simulink model "PSAS_Rocket_sim"  (R2013a)
settings: Solver=ode45  StartTime=0.0  StopTime=10.0  RelTol=1e-3
values from neighbouring files (symbols this model uses):
  burn = 0.25    [PSAS_Rocket_sys.m]    (also in stevens_state_space_for_rocket.m)
  burntime = m_fuel/burn    (= 40)    [PSAS_Rocket_sys.m]    (also in stevens_state_space_for_rocket.m = 76)
  F_pitch = 5.5    [PSAS_Rocket_sys.m]
  F_roll = 7    [PSAS_Rocket_sys.m]
  F_yaw = 5.5    [PSAS_Rocket_sys.m]
  g = 9.81    [PSAS_Rocket_sys.m]    (also in stevens_state_space_for_rocket.m)
  hz = 5    [PSAS_Rocket_sys.m]    (also in roll_sys.m; rotational_system.m = 10)
  Inertia = [Ixx -Ixy -Ixz; -Ixy Iyy -Iyz; -Ixz -Iyz Izz]    [PSAS_Rocket_sys.m]
  Ixx = .05    (= 0.05)    [PSAS_Rocket_sys.m]
  Ixy = 0.02    [PSAS_Rocket_sys.m]
  Ixz = 0.05    [PSAS_Rocket_sys.m]
  Iyy = .05    (= 0.05)    [PSAS_Rocket_sys.m]
  Iyz = 0.02    [PSAS_Rocket_sys.m]
  Izz = 0.0169    [PSAS_Rocket_sys.m]
  kp_phi = .001    (= 0.001)    [PSAS_Rocket_sys.m]
  kp_psi = .2    (= 0.2)    [PSAS_Rocket_sys.m]
  kp_theta = .001    (= 0.001)    [PSAS_Rocket_sys.m]
  m_fuel = 10    [PSAS_Rocket_sys.m]    (also in stevens_state_space_for_rocket.m = 19)
  m_inst = 3    [PSAS_Rocket_sys.m]    (also in stevens_state_space_for_rocket.m = 3.8)
  q1 = cos(psi/2)*cos(theta/2)*cos(phi/2)     + sin(psi/2)*sin(theta/2)*sin(phi/2)    [PSAS_Rocket_sys.m]    (also in stevens_state_space_for_rocket.m = sin(phi/2)*cos(theta/2)*cos(psi/2)-cos(phi/2)*     sin(theta)
  q2 = cos(psi/2)*cos(theta/2)*sin(phi/2)     - sin(psi/2)*sin(theta/2)*cos(phi/2)    [PSAS_Rocket_sys.m]    (also in stevens_state_space_for_rocket.m = cos(phi/2)*sin(theta/2)*cos(psi/2)+sin(phi/2)*     cos(theta)
  q3 = cos(psi/2)*sin(theta/2)*cos(phi/2)     + sin(psi/2)*cos(theta/2)*sin(phi/2)    [PSAS_Rocket_sys.m]    (also in stevens_state_space_for_rocket.m = cos(phi/2)*cos(theta/2)*sin(psi/2)-sin(phi/2)*     sin(theta)
  q4 = sin(psi/2)*cos(theta/2)*cos(phi/2)     - cos(psi/2)*sin(theta/2)*sin(phi/2)    [PSAS_Rocket_sys.m]
  roll_disturbance = 1*pi/180    (= 0.0174532925199)    [PSAS_Rocket_sys.m]
  tau = 0.02    [PSAS_Rocket_sys.m]    (also in lqrQfinder.m = 0.009; stevens_state_space_for_rocket.m = 0.05)
  theta_in = 90*pi/180    (= 1.57079632679)    [PSAS_Rocket_sys.m]
  theta_in_ramp = 2    [PSAS_Rocket_sys.m]
  thrust = 4440.8    [PSAS_Rocket_sys.m]    (also in stevens_state_space_for_rocket.m = 444.8)
  thrust_lag = 1.5    [PSAS_Rocket_sys.m]
  ts = .003    (= 0.003)    [PSAS_Rocket_sys.m]    (also in stevens_state_space_for_rocket.m = 0.01)
libraries: simulink x8
settings Model: Creator=kenny  LastModifiedBy=kenny

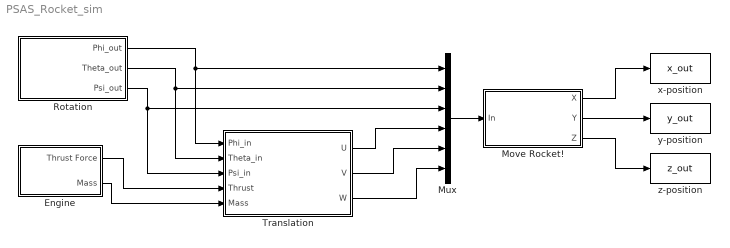
== system PSAS_Rocket_sim ==
  Engine : Subsystem
  Move Rocket! : Subsystem
  Mux : Mux  Inputs=6
  Rotation : Subsystem
  Translation : Subsystem
  x-position : ToWorkspace  VariableName=x_out  SampleTime=-1  SaveFormat=Structure With Time
  y-position : ToWorkspace  VariableName=y_out  SampleTime=-1  SaveFormat=Structure With Time
  z-position : ToWorkspace  VariableName=z_out  SampleTime=-1  SaveFormat=Structure With Time
  wires:
  Rotation/1(Phi_out) -> Translation/1(Phi_in), Mux/1
  Rotation/2(Theta_out) -> Translation/2(Theta_in), Mux/2
  Rotation/3(Psi_out) -> Translation/3(Psi_in), Mux/3
  Translation/2(V) -> Mux/5
  Translation/3(W) -> Mux/6
  Translation/1(U) -> Mux/4
  Engine/1(Thrust Force) -> Translation/4(Thrust)
  Engine/2(Mass) -> Translation/5(Mass)
  Mux/1 -> Move Rocket!/1(In)
  Move Rocket!/2(Y) -> y-position/1
  Move Rocket!/1(X) -> x-position/1
  Move Rocket!/3(Z) -> z-position/1

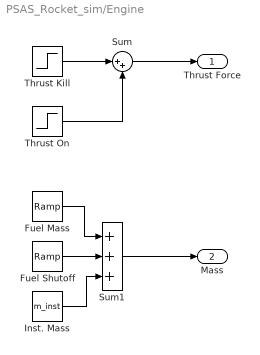
== system PSAS_Rocket_sim/Engine ==
  Fuel Mass : simulink/Sources/Ramp  slope=-burn  start=0  X0=m_fuel
  Fuel Shutoff : simulink/Sources/Ramp  slope=burn  start=burntime  X0=0
  Inst. Mass : Constant  Value=m_inst
  Sum : Sum  Inputs=|++
  Sum1 : Sum  Inputs=+++
  Thrust Kill : Step  Time=burntime+thrust_lag  After=-thrust  SampleTime=0
  Thrust On : Step  Time=thrust_lag  After=thrust  SampleTime=0
  Thrust Force : Outport
  Mass : Outport  Port=2
  wires:
  Thrust Kill/1 -> Sum/1
  Thrust On/1 -> Sum/2
  Sum/1 -> Thrust Force/1
  Sum1/1 -> Mass/1
  Fuel Mass/1 -> Sum1/1
  Fuel Shutoff/1 -> Sum1/2
  Inst. Mass/1 -> Sum1/3

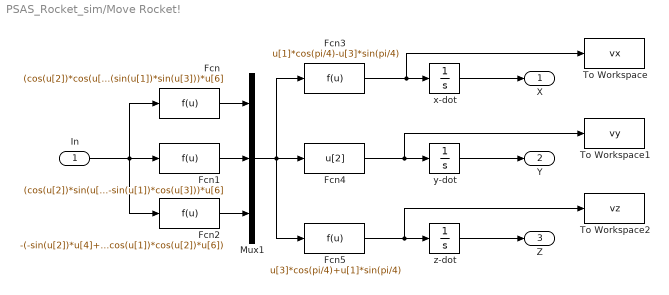
== system PSAS_Rocket_sim/Move Rocket! ==
  In : Inport
  Fcn : Fcn  Expr=(cos(u[2])*cos(u[3]))*u[4]+(sin(u[1])*sin(u[2])*cos(u[3])-cos(u[1])*sin(u[3]))*u[5]+(sin(u[1])*sin(u[3]))*u[6]
  Fcn1 : Fcn  Expr=(cos(u[2])*sin(u[3]))*u[4]+(sin(u[1])*sin(u[2])*sin(u[3])+cos(u[1])*cos(u[3]))*u[5]+(cos(u[1])*sin(u[2])*sin(u[3])-sin(u[1])*cos(u[3]))*u[6]
  Fcn2 : Fcn  Expr=-(-sin(u[2])*u[4]+sin(u[1])*cos(u[2])*u[5]+cos(u[1])*cos(u[2])*u[6])
  Fcn3 : Fcn  Expr=u[1]*cos(pi/4)-u[3]*sin(pi/4)
  Fcn4 : Fcn  Expr=u[2]
  Fcn5 : Fcn  Expr=u[3]*cos(pi/4)+u[1]*sin(pi/4)
  Mux1 : Mux  Inputs=3
  To Workspace : ToWorkspace  VariableName=vx  SampleTime=-1
  To Workspace1 : ToWorkspace  VariableName=vy  SampleTime=-1
  To Workspace2 : ToWorkspace  VariableName=vz  SampleTime=-1
  x-dot : Integrator
  y-dot : Integrator
  z-dot : Integrator
  X : Outport
  Y : Outport  Port=2
  Z : Outport  Port=3
  wires:
  In/1 -> Fcn/1, Fcn2/1, Fcn1/1
  z-dot/1 -> Z/1
  y-dot/1 -> Y/1
  x-dot/1 -> X/1
  Fcn/1 -> Mux1/1
  Fcn1/1 -> Mux1/2
  Fcn2/1 -> Mux1/3
  Mux1/1 -> Fcn4/1, Fcn3/1, Fcn5/1
  Fcn3/1 -> To Workspace/1, x-dot/1
  Fcn4/1 -> y-dot/1, To Workspace1/1
  Fcn5/1 -> z-dot/1, To Workspace2/1

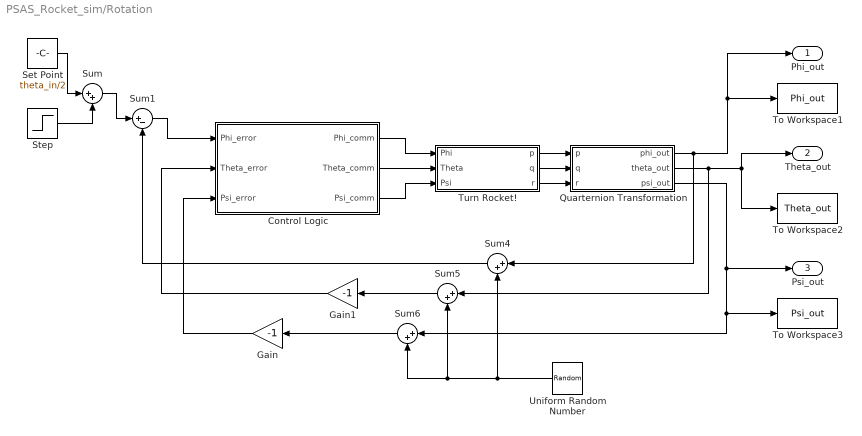
== system PSAS_Rocket_sim/Rotation ==
  Control Logic : Subsystem
  Gain : Gain  Gain=-1
  Gain1 : Gain  Gain=-1
  Quarternion Transformation : Subsystem
  Set Point : Constant  Value=theta_in/2
  Step : Step  Time=theta_in_ramp  After=theta_in/2  SampleTime=0
  Sum{,4..6} (4 alike) : Sum  Inputs=|++
  Sum1 : Sum  Inputs=|+-
  To Workspace1 : ToWorkspace  VariableName=Phi_out  SampleTime=-1  SaveFormat=Structure With Time
  To Workspace2 : ToWorkspace  VariableName=Theta_out  SampleTime=-1  SaveFormat=Structure With Time
  To Workspace3 : ToWorkspace  VariableName=Psi_out  SampleTime=-1  SaveFormat=Structure With Time
  Turn Rocket! : Subsystem
  Uniform Random Number : UniformRandomNumber  Minimum=-roll_disturbance  Maximum=roll_disturbance  SampleTime=ts
  Phi_out : Outport
  Theta_out : Outport  Port=2
  Psi_out : Outport  Port=3
  wires:
  Step/1 -> Sum/2
  Set Point/1 -> Sum/1
  Sum/1 -> Sum1/1
  Control Logic/1(Phi_comm) -> Turn Rocket!/1(Phi)
  Control Logic/2(Theta_comm) -> Turn Rocket!/2(Theta)
  Control Logic/3(Psi_comm) -> Turn Rocket!/3(Psi)
  Turn Rocket!/1(p) -> Quarternion Transformation/1(p)
  Turn Rocket!/2(q) -> Quarternion Transformation/2(q)
  Turn Rocket!/3(r) -> Quarternion Transformation/3(r)
  Quarternion Transformation/2(theta_out) -> Sum5/1, To Workspace2/1, Theta_out/1
  Quarternion Transformation/1(phi_out) -> Sum4/1, Phi_out/1, To Workspace1/1
  Quarternion Transformation/3(psi_out) -> Sum6/1, To Workspace3/1, Psi_out/1
  Uniform Random Number/1 -> Sum6/2, Sum5/2, Sum4/2
  Sum6/1 -> Gain/1
  Sum5/1 -> Gain1/1
  Gain/1 -> Control Logic/3(Psi_error)
  Gain1/1 -> Control Logic/2(Theta_error)
  Sum1/1 -> Control Logic/1(Phi_error)
  Sum4/1 -> Sum1/2

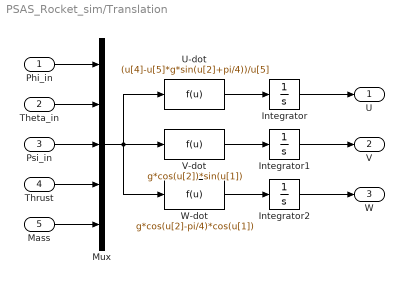
== system PSAS_Rocket_sim/Translation ==
  Phi_in : Inport
  Theta_in : Inport  Port=2
  Psi_in : Inport  Port=3
  Thrust : Inport  Port=4
  Mass : Inport  Port=5
  Integrator : Integrator
  Integrator1 : Integrator
  Integrator2 : Integrator
  Mux : Mux  Inputs=5
  U-dot : Fcn  Expr=(u[4]-u[5]*g*sin(u[2]+pi/4))/u[5]
  V-dot : Fcn  Expr=g*cos(u[2])*sin(u[1])
  W-dot : Fcn  Expr=g*cos(u[2]-pi/4)*cos(u[1])
  U : Outport
  V : Outport  Port=2
  W : Outport  Port=3
  wires:
  Phi_in/1 -> Mux/1
  Theta_in/1 -> Mux/2
  Psi_in/1 -> Mux/3
  U-dot/1 -> Integrator/1
  Mux/1 -> U-dot/1, V-dot/1, W-dot/1
  V-dot/1 -> Integrator1/1
  W-dot/1 -> Integrator2/1
  Thrust/1 -> Mux/4
  Mass/1 -> Mux/5
  Integrator/1 -> U/1
  Integrator1/1 -> V/1
  Integrator2/1 -> W/1

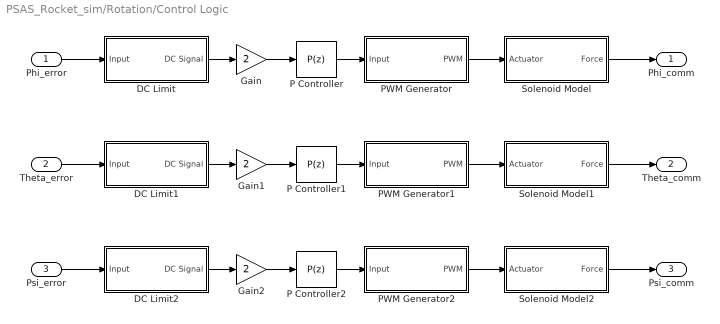
== system PSAS_Rocket_sim/Rotation/Control Logic ==
  Phi_error : Inport
  Theta_error : Inport  Port=2
  Psi_error : Inport  Port=3
  DC Limit : Subsystem
  DC Limit1 : Subsystem
  DC Limit2 : Subsystem
  Gain : Gain  Gain=2
  Gain1 : Gain  Gain=2
  Gain2 : Gain  Gain=2
  P Controller : simulink/Continuous/PID Controller  Controller=P  TimeDomain=Discrete-time  SampleTime=ts  IntegratorMethod=Forward Euler  FilterMethod=Forward Euler  Form=Parallel  P=kp_phi  I=0  D=0  N=100  InitialConditionSource=internal  InitialConditionForIntegrator=0  InitialConditionForFilter=0  ExternalReset=none  LimitOutput=off  UpperSaturationLimit=inf  LowerSaturationLimit=-inf  LinearizeAsGain=on  AntiWindupMode=none  Kb=1  TrackingMode=off  Kt=1  PParamMin=[]  PParamMax=[]  IParamMin=[]  IParamMax=[]  DParamMin=[]  DParamMax=[]  NParamMin=[]  NParamMax=[]  KbParamMin=[]  KbParamMax=[]  KtParamMin=[]  KtParamMax=[]  POutMin=[]  POutMax=[]  IOutMin=[]  IOutMax=[]  DOutMin=[]  DOutMax=[]  NOutMin=[]  NOutMax=[]  KbOutMin=[]  KbOutMax=[]  KtOutMin=[]  KtOutMax=[]  IntegratorOutMin=[]  IntegratorOutMax=[]  FilterOutMin=[]  FilterOutMax=[]  SumOutMin=[]  SumOutMax=[]  SumI1OutMin=[]  SumI1OutMax=[]  SumI2OutMin=[]  SumI2OutMax=[]  SumI3OutMin=[]  SumI3OutMax=[]  SumDOutMin=[]  SumDOutMax=[]  SaturationOutMin=[]  SaturationOutMax=[]  IntegratorContinuousStateAttributes=''  IntegratorStateMustResolveToSignalObject=off  IntegratorRTWStateStorageClass=Auto  FilterContinuousStateAttributes=''  FilterStateMustResolveToSignalObject=off  FilterRTWStateStorageClass=Auto
  P Controller1 : simulink/Continuous/PID Controller  Controller=P  TimeDomain=Discrete-time  SampleTime=ts  IntegratorMethod=Forward Euler  FilterMethod=Forward Euler  Form=Parallel  P=kp_theta  I=0  D=0  N=100  InitialConditionSource=internal  InitialConditionForIntegrator=0  InitialConditionForFilter=0  ExternalReset=none  LimitOutput=off  UpperSaturationLimit=inf  LowerSaturationLimit=-inf  LinearizeAsGain=on  AntiWindupMode=none  Kb=1  TrackingMode=off  Kt=1  PParamMin=[]  PParamMax=[]  IParamMin=[]  IParamMax=[]  DParamMin=[]  DParamMax=[]  NParamMin=[]  NParamMax=[]  KbParamMin=[]  KbParamMax=[]  KtParamMin=[]  KtParamMax=[]  POutMin=[]  POutMax=[]  IOutMin=[]  IOutMax=[]  DOutMin=[]  DOutMax=[]  NOutMin=[]  NOutMax=[]  KbOutMin=[]  KbOutMax=[]  KtOutMin=[]  KtOutMax=[]  IntegratorOutMin=[]  IntegratorOutMax=[]  FilterOutMin=[]  FilterOutMax=[]  SumOutMin=[]  SumOutMax=[]  SumI1OutMin=[]  SumI1OutMax=[]  SumI2OutMin=[]  SumI2OutMax=[]  SumI3OutMin=[]  SumI3OutMax=[]  SumDOutMin=[]  SumDOutMax=[]  SaturationOutMin=[]  SaturationOutMax=[]  IntegratorContinuousStateAttributes=''  IntegratorStateMustResolveToSignalObject=off  IntegratorRTWStateStorageClass=Auto  FilterContinuousStateAttributes=''  FilterStateMustResolveToSignalObject=off  FilterRTWStateStorageClass=Auto
  P Controller2 : simulink/Continuous/PID Controller  Controller=P  TimeDomain=Discrete-time  SampleTime=ts  IntegratorMethod=Forward Euler  FilterMethod=Forward Euler  Form=Parallel  P=kp_psi  I=0  D=0  N=100  InitialConditionSource=internal  InitialConditionForIntegrator=0  InitialConditionForFilter=0  ExternalReset=none  LimitOutput=off  UpperSaturationLimit=inf  LowerSaturationLimit=-inf  LinearizeAsGain=on  AntiWindupMode=none  Kb=1  TrackingMode=off  Kt=1  PParamMin=[]  PParamMax=[]  IParamMin=[]  IParamMax=[]  DParamMin=[]  DParamMax=[]  NParamMin=[]  NParamMax=[]  KbParamMin=[]  KbParamMax=[]  KtParamMin=[]  KtParamMax=[]  POutMin=[]  POutMax=[]  IOutMin=[]  IOutMax=[]  DOutMin=[]  DOutMax=[]  NOutMin=[]  NOutMax=[]  KbOutMin=[]  KbOutMax=[]  KtOutMin=[]  KtOutMax=[]  IntegratorOutMin=[]  IntegratorOutMax=[]  FilterOutMin=[]  FilterOutMax=[]  SumOutMin=[]  SumOutMax=[]  SumI1OutMin=[]  SumI1OutMax=[]  SumI2OutMin=[]  SumI2OutMax=[]  SumI3OutMin=[]  SumI3OutMax=[]  SumDOutMin=[]  SumDOutMax=[]  SaturationOutMin=[]  SaturationOutMax=[]  IntegratorContinuousStateAttributes=''  IntegratorStateMustResolveToSignalObject=off  IntegratorRTWStateStorageClass=Auto  FilterContinuousStateAttributes=''  FilterStateMustResolveToSignalObject=off  FilterRTWStateStorageClass=Auto
  PWM Generator : Subsystem
  PWM Generator1 : Subsystem
  PWM Generator2 : Subsystem
  Solenoid Model : Subsystem
  Solenoid Model1 : Subsystem
  Solenoid Model2 : Subsystem
  Phi_comm : Outport
  Theta_comm : Outport  Port=2
  Psi_comm : Outport  Port=3
  wires:
  PWM Generator/1(PWM) -> Solenoid Model/1(Actuator)
  P Controller/1 -> PWM Generator/1(Input)
  Solenoid Model/1(Force) -> Phi_comm/1
  PWM Generator1/1(PWM) -> Solenoid Model1/1(Actuator)
  P Controller1/1 -> PWM Generator1/1(Input)
  Solenoid Model1/1(Force) -> Theta_comm/1
  PWM Generator2/1(PWM) -> Solenoid Model2/1(Actuator)
  P Controller2/1 -> PWM Generator2/1(Input)
  Solenoid Model2/1(Force) -> Psi_comm/1
  Phi_error/1 -> DC Limit/1(Input)
  Theta_error/1 -> DC Limit1/1(Input)
  Psi_error/1 -> DC Limit2/1(Input)
  DC Limit/1(DC Signal) -> Gain/1
  Gain/1 -> P Controller/1
  DC Limit1/1(DC Signal) -> Gain1/1
  Gain1/1 -> P Controller1/1
  DC Limit2/1(DC Signal) -> Gain2/1
  Gain2/1 -> P Controller2/1

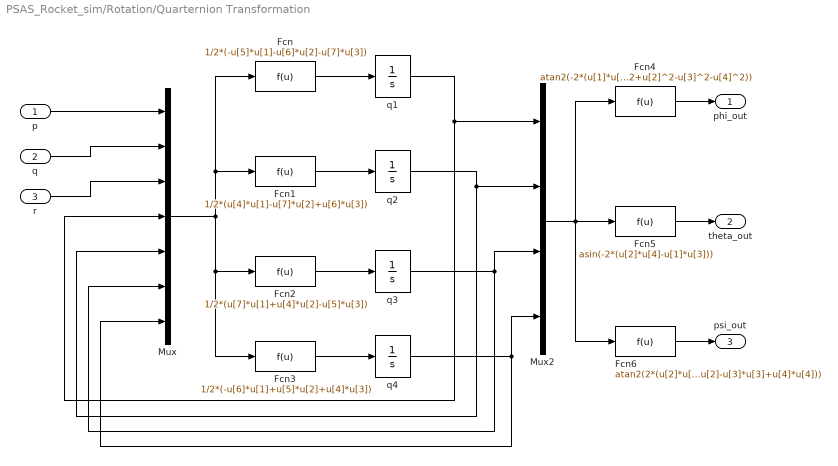
== system PSAS_Rocket_sim/Rotation/Quarternion Transformation ==
  p : Inport
  q : Inport  Port=2
  r : Inport  Port=3
  Fcn : Fcn  Expr=1/2*(-u[5]*u[1]-u[6]*u[2]-u[7]*u[3])
  Fcn1 : Fcn  Expr=1/2*(u[4]*u[1]-u[7]*u[2]+u[6]*u[3])
  Fcn2 : Fcn  Expr=1/2*(u[7]*u[1]+u[4]*u[2]-u[5]*u[3])
  Fcn3 : Fcn  Expr=1/2*(-u[6]*u[1]+u[5]*u[2]+u[4]*u[3])
  Fcn4 : Fcn  Expr=atan2(-2*(u[1]*u[2]+u[3]*u[4]),(u[1]^2+u[2]^2-u[3]^2-u[4]^2))
  Fcn5 : Fcn  Expr=asin(-2*(u[2]*u[4]-u[1]*u[3]))
  Fcn6 : Fcn  Expr=atan2(2*(u[2]*u[3]+u[1]*u[4]),(u[1]*u[1]-u[2]*u[2]-u[3]*u[3]+u[4]*u[4]))
  Mux : Mux  Inputs=7
  Mux2 : Mux
  q1 : Integrator  InitialCondition=q1
  q2 : Integrator  InitialCondition=q2
  q3 : Integrator  InitialCondition=q3
  q4 : Integrator  InitialCondition=q4
  phi_out : Outport
  theta_out : Outport  Port=2
  psi_out : Outport  Port=3
  wires:
  p/1 -> Mux/1
  q/1 -> Mux/2
  r/1 -> Mux/3
  q1/1 -> Mux/4, Mux2/1
  q2/1 -> Mux/5, Mux2/2
  q3/1 -> Mux2/3, Mux/6
  q4/1 -> Mux2/4, Mux/7
  Mux/1 -> Fcn/1, Fcn1/1, Fcn3/1, Fcn2/1
  Fcn/1 -> q1/1
  Fcn1/1 -> q2/1
  Fcn2/1 -> q3/1
  Fcn3/1 -> q4/1
  Mux2/1 -> Fcn6/1, Fcn5/1, Fcn4/1
  Fcn4/1 -> phi_out/1
  Fcn5/1 -> theta_out/1
  Fcn6/1 -> psi_out/1

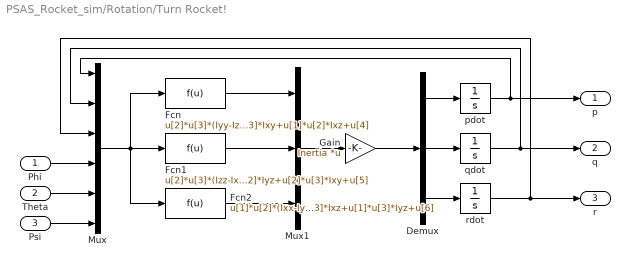
== system PSAS_Rocket_sim/Rotation/Turn Rocket! ==
  Phi : Inport
  Theta : Inport  Port=2
  Psi : Inport  Port=3
  Demux : Demux  Outputs=3
  Fcn : Fcn  Expr=u[2]*u[3]*(Iyy-Izz)+(u[2]^2-u[3]^2)*Iyz-u[1]*u[3]*Ixy+u[1]*u[2]*Ixz+u[4]
  Fcn1 : Fcn  Expr=u[2]*u[3]*(Izz-Ixx)+(u[3]^2-u[1]^2)*Ixz-u[1]*u[2]*Iyz+u[2]*u[3]*Ixy+u[5]
  Fcn2 : Fcn  Expr=u[1]*u[2]*(Ixx-Iyy)+(u[1]^2-u[2]^2)*Ixy-u[2]*u[3]*Ixz+u[1]*u[3]*Iyz+u[6]
  Gain : Gain  Gain=Inertia  Multiplication=Matrix(K*u)
  Mux : Mux  Inputs=6
  Mux1 : Mux  Inputs=3
  pdot : Integrator
  qdot : Integrator
  rdot : Integrator
  p : Outport
  q : Outport  Port=2
  r : Outport  Port=3
  wires:
  rdot/1 -> r/1, Mux/3
  qdot/1 -> q/1, Mux/2
  pdot/1 -> p/1, Mux/1
  Phi/1 -> Mux/4
  Theta/1 -> Mux/5
  Demux/1 -> pdot/1
  Demux/2 -> qdot/1
  Demux/3 -> rdot/1
  Gain/1 -> Demux/1
  Mux1/1 -> Gain/1
  Fcn/1 -> Mux1/1
  Fcn1/1 -> Mux1/2
  Fcn2/1 -> Mux1/3
  Mux/1 -> Fcn1/1, Fcn/1, Fcn2/1
  Psi/1 -> Mux/6

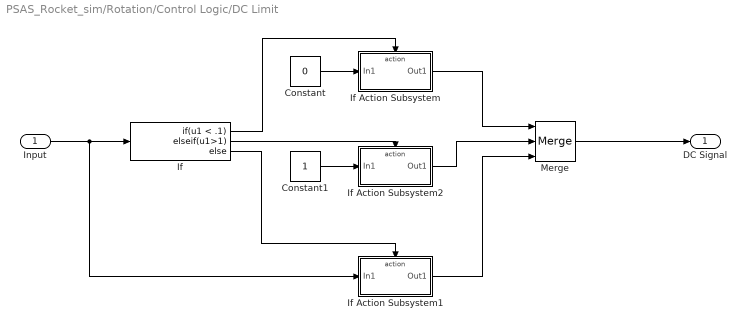
== system PSAS_Rocket_sim/Rotation/Control Logic/DC Limit ==
  Input : Inport
  Constant : Constant  Value=0
  Constant1 : Constant
  If : If  IfExpression=u1 < .1  ElseIfExpressions=u1>1
  If Action Subsystem : Subsystem  TreatAsAtomicUnit=on
  If Action Subsystem1 : Subsystem  TreatAsAtomicUnit=on
  If Action Subsystem2 : Subsystem  TreatAsAtomicUnit=on
  Merge : Merge  Inputs=3
  DC Signal : Outport
  wires:
  Input/1 -> If Action Subsystem1/1(In1), If/1
  Merge/1 -> DC Signal/1
  If Action Subsystem/1(Out1) -> Merge/1
  Constant/1 -> If Action Subsystem/1(In1)
  If/1 -> If Action Subsystem/Action
  If/3 -> If Action Subsystem1/Action
  If Action Subsystem1/1(Out1) -> Merge/3
  If/2 -> If Action Subsystem2/Action
  If Action Subsystem2/1(Out1) -> Merge/2
  Constant1/1 -> If Action Subsystem2/1(In1)

== system PSAS_Rocket_sim/Rotation/Control Logic/DC Limit1 ==
  Input : Inport
  Constant : Constant  Value=0
  Constant1 : Constant
  If : If  IfExpression=u1 < .1  ElseIfExpressions=u1>1
  If Action Subsystem : Subsystem  TreatAsAtomicUnit=on
  If Action Subsystem1 : Subsystem  TreatAsAtomicUnit=on
  If Action Subsystem2 : Subsystem  TreatAsAtomicUnit=on
  Merge : Merge  Inputs=3
  DC Signal : Outport
  wires:
  Constant1/1 -> If Action Subsystem2/1(In1)
  If Action Subsystem2/1(Out1) -> Merge/2
  If/2 -> If Action Subsystem2/Action
  If Action Subsystem1/1(Out1) -> Merge/3
  If/3 -> If Action Subsystem1/Action
  If/1 -> If Action Subsystem/Action
  Constant/1 -> If Action Subsystem/1(In1)
  If Action Subsystem/1(Out1) -> Merge/1
  Merge/1 -> DC Signal/1
  Input/1 -> If/1, If Action Subsystem1/1(In1)

== system PSAS_Rocket_sim/Rotation/Control Logic/DC Limit2 ==
  Input : Inport
  Constant : Constant  Value=0
  Constant1 : Constant
  If : If  IfExpression=u1 < .1  ElseIfExpressions=u1>1
  If Action Subsystem : Subsystem  TreatAsAtomicUnit=on
  If Action Subsystem1 : Subsystem  TreatAsAtomicUnit=on
  If Action Subsystem2 : Subsystem  TreatAsAtomicUnit=on
  Merge : Merge  Inputs=3
  DC Signal : Outport
  wires:
  Input/1 -> If Action Subsystem1/1(In1), If/1
  Merge/1 -> DC Signal/1
  If Action Subsystem/1(Out1) -> Merge/1
  Constant/1 -> If Action Subsystem/1(In1)
  If/1 -> If Action Subsystem/Action
  If/3 -> If Action Subsystem1/Action
  If Action Subsystem1/1(Out1) -> Merge/3
  If/2 -> If Action Subsystem2/Action
  If Action Subsystem2/1(Out1) -> Merge/2
  Constant1/1 -> If Action Subsystem2/1(In1)

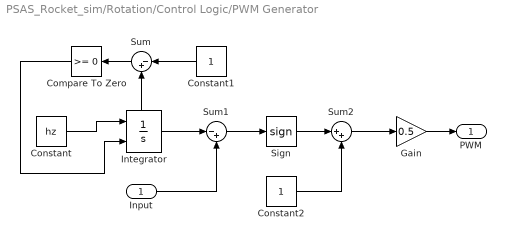
== system PSAS_Rocket_sim/Rotation/Control Logic/PWM Generator ==
  Input : Inport
  Compare To Zero : simulink/Logic and Bit Operations/Compare To Zero  relop=>=  OutDataTypeStr=boolean
  Constant : Constant  Value=hz
  Constant1 : Constant
  Constant2 : Constant
  Gain : Gain  Gain=0.5
  Integrator : Integrator  ExternalReset=rising  ShowStatePort=on
  Sign : Signum
  Sum : Sum  Inputs=|-+
  Sum1 : Sum  Inputs=|-+
  Sum2 : Sum  Inputs=|++
  PWM : Outport
  wires:
  Constant1/1 -> Sum/1
  Sum/1 -> Compare To Zero/1
  Integrator/1 -> Sum1/1
  Input/1 -> Sum1/2
  Sum1/1 -> Sign/1
  Sign/1 -> Sum2/1
  Constant2/1 -> Sum2/2
  Sum2/1 -> Gain/1
  Gain/1 -> PWM/1
  Constant/1 -> Integrator/1
  Compare To Zero/1 -> Integrator/2
  Integrator/State -> Sum/2

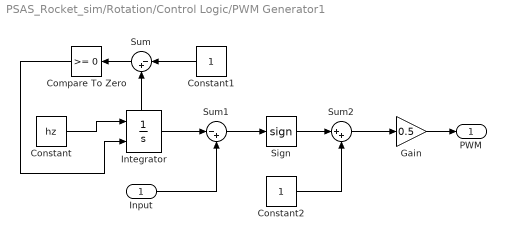
== system PSAS_Rocket_sim/Rotation/Control Logic/PWM Generator1 ==
  Input : Inport
  Compare To Zero : simulink/Logic and Bit Operations/Compare To Zero  relop=>=  OutDataTypeStr=boolean
  Constant : Constant  Value=hz
  Constant1 : Constant
  Constant2 : Constant
  Gain : Gain  Gain=0.5
  Integrator : Integrator  ExternalReset=rising  ShowStatePort=on
  Sign : Signum
  Sum : Sum  Inputs=|-+
  Sum1 : Sum  Inputs=|-+
  Sum2 : Sum  Inputs=|++
  PWM : Outport
  wires:
  Integrator/State -> Sum/2
  Compare To Zero/1 -> Integrator/2
  Constant/1 -> Integrator/1
  Gain/1 -> PWM/1
  Sum2/1 -> Gain/1
  Constant2/1 -> Sum2/2
  Sign/1 -> Sum2/1
  Sum1/1 -> Sign/1
  Input/1 -> Sum1/2
  Integrator/1 -> Sum1/1
  Sum/1 -> Compare To Zero/1
  Constant1/1 -> Sum/1

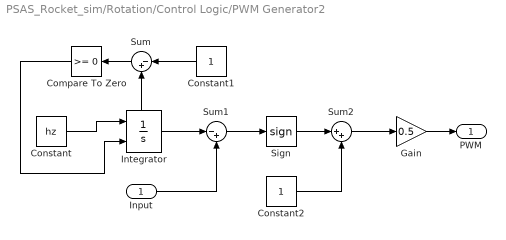
== system PSAS_Rocket_sim/Rotation/Control Logic/PWM Generator2 ==
  Input : Inport
  Compare To Zero : simulink/Logic and Bit Operations/Compare To Zero  relop=>=  OutDataTypeStr=boolean
  Constant : Constant  Value=hz
  Constant1 : Constant
  Constant2 : Constant
  Gain : Gain  Gain=0.5
  Integrator : Integrator  ExternalReset=rising  ShowStatePort=on
  Sign : Signum
  Sum : Sum  Inputs=|-+
  Sum1 : Sum  Inputs=|-+
  Sum2 : Sum  Inputs=|++
  PWM : Outport
  wires:
  Constant1/1 -> Sum/1
  Sum/1 -> Compare To Zero/1
  Integrator/1 -> Sum1/1
  Input/1 -> Sum1/2
  Sum1/1 -> Sign/1
  Sign/1 -> Sum2/1
  Constant2/1 -> Sum2/2
  Sum2/1 -> Gain/1
  Gain/1 -> PWM/1
  Constant/1 -> Integrator/1
  Compare To Zero/1 -> Integrator/2
  Integrator/State -> Sum/2

== system PSAS_Rocket_sim/Rotation/Control Logic/Solenoid Model ==
  Actuator : Inport
  Data Type Conversion : DataTypeConversion
  Gain : Gain  Gain=F_roll
  Saturation : Saturate  UpperLimit=F_roll  LowerLimit=-F_roll
  Solenoid Transfer Fcn : TransferFcn  Denominator=[tau 1]
  Force : Outport
  wires:
  Gain/1 -> Solenoid Transfer Fcn/1
  Saturation/1 -> Force/1
  Data Type Conversion/1 -> Gain/1
  Solenoid Transfer Fcn/1 -> Saturation/1
  Actuator/1 -> Data Type Conversion/1

== system PSAS_Rocket_sim/Rotation/Control Logic/Solenoid Model1 ==
  Actuator : Inport
  Data Type Conversion : DataTypeConversion
  Gain : Gain  Gain=F_pitch
  Saturation : Saturate  UpperLimit=F_pitch  LowerLimit=-F_pitch
  Solenoid Transfer Fcn : TransferFcn  Denominator=[tau 1]
  Force : Outport
  wires:
  Actuator/1 -> Data Type Conversion/1
  Solenoid Transfer Fcn/1 -> Saturation/1
  Data Type Conversion/1 -> Gain/1
  Saturation/1 -> Force/1
  Gain/1 -> Solenoid Transfer Fcn/1

== system PSAS_Rocket_sim/Rotation/Control Logic/Solenoid Model2 ==
  Actuator : Inport
  Data Type Conversion : DataTypeConversion
  Gain : Gain  Gain=F_yaw
  Saturation : Saturate  UpperLimit=F_yaw  LowerLimit=-F_yaw
  Solenoid Transfer Fcn : TransferFcn  Denominator=[tau 1]
  Force : Outport
  wires:
  Gain/1 -> Solenoid Transfer Fcn/1
  Saturation/1 -> Force/1
  Data Type Conversion/1 -> Gain/1
  Solenoid Transfer Fcn/1 -> Saturation/1
  Actuator/1 -> Data Type Conversion/1

== system PSAS_Rocket_sim/Rotation/Control Logic/DC Limit/If Action Subsystem ==
  In1 : Inport
  Action Port : ActionPort  ActionType=then
  Out1 : Outport
  wires:
  In1/1 -> Out1/1

== system PSAS_Rocket_sim/Rotation/Control Logic/DC Limit/If Action Subsystem1 ==
  In1 : Inport
  Action Port : ActionPort  ActionType=else
  Out1 : Outport
  wires:
  In1/1 -> Out1/1

== system PSAS_Rocket_sim/Rotation/Control Logic/DC Limit/If Action Subsystem2 ==
  In1 : Inport
  Action Port : ActionPort  ActionType=elseif
  Out1 : Outport
  wires:
  In1/1 -> Out1/1

== system PSAS_Rocket_sim/Rotation/Control Logic/DC Limit1/If Action Subsystem ==
  In1 : Inport
  Action Port : ActionPort  ActionType=then
  Out1 : Outport
  wires:
  In1/1 -> Out1/1

== system PSAS_Rocket_sim/Rotation/Control Logic/DC Limit1/If Action Subsystem1 ==
  In1 : Inport
  Action Port : ActionPort  ActionType=else
  Out1 : Outport
  wires:
  In1/1 -> Out1/1

== system PSAS_Rocket_sim/Rotation/Control Logic/DC Limit1/If Action Subsystem2 ==
  In1 : Inport
  Action Port : ActionPort  ActionType=elseif
  Out1 : Outport
  wires:
  In1/1 -> Out1/1

== system PSAS_Rocket_sim/Rotation/Control Logic/DC Limit2/If Action Subsystem ==
  In1 : Inport
  Action Port : ActionPort  ActionType=then
  Out1 : Outport
  wires:
  In1/1 -> Out1/1

== system PSAS_Rocket_sim/Rotation/Control Logic/DC Limit2/If Action Subsystem1 ==
  In1 : Inport
  Action Port : ActionPort  ActionType=else
  Out1 : Outport
  wires:
  In1/1 -> Out1/1

== system PSAS_Rocket_sim/Rotation/Control Logic/DC Limit2/If Action Subsystem2 ==
  In1 : Inport
  Action Port : ActionPort  ActionType=elseif
  Out1 : Outport
  wires:
  In1/1 -> Out1/1
